simulink model "One_Press_ChangeState"  (R2024a)
settings: Solver=VariableStepAuto  StartTime=0.0  StopTime=10.0  RelTol=1e-3
libraries: arduinolib x2, simulink x1
settings Model: Creator=VICTUS  LastModifiedBy=VICTUS

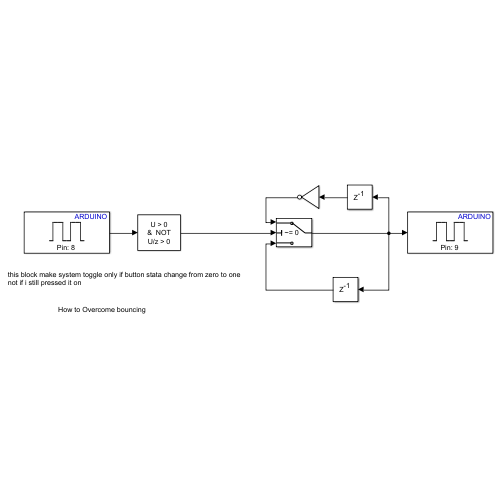
[thumbnail: Simulink's stored preview of the top-level diagram]
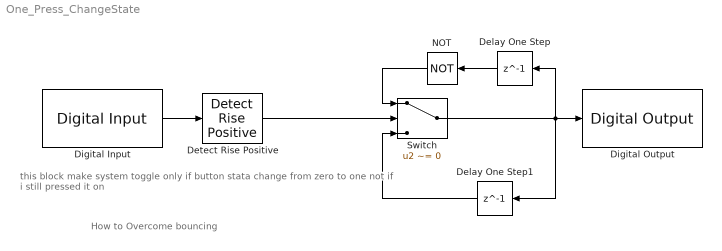
== system One_Press_ChangeState ==
  note: this block make system toggle only if button stata change from zero to one not if i still pressed it on
  note: How to Overcome bouncing
  Delay One Step : Delay  DelayLength=1
  Delay One Step1 : Delay  DelayLength=1
  Detect Rise Positive : simulink/Logic and Bit Operations/Detect Rise Positive  vinit=0  OutDataTypeStr=boolean
  Digital Input : arduinolib/Digital Input  pinNumber=8  mode=Default  Direction=input  SampleTime=0.1  blockPlatform=arduino
  Digital Output : arduinolib/Digital Output  pinNumber=9  Direction=output  blockPlatform=arduino
  NOT : Logic  Operator=NOT  IconShape=distinctive  AllPortsSameDT=off  OutDataTypeStr=boolean
  Switch : Switch  Criteria=u2 ~= 0  SaturateOnIntegerOverflow=off  InputSameDT=off
  wires:
  Digital Input/1 -> Detect Rise Positive/1
  Detect Rise Positive/1 -> Switch/2
  Switch/1 -> Delay One Step/1, Delay One Step1/1, Digital Output/1
  Delay One Step1/1 -> Switch/3
  Delay One Step/1 -> NOT/1
  NOT/1 -> Switch/1
